simulink model "PTC_MBDS_ScrollCenteredNoWrap_Sample"  (R2013a)
settings: Solver=VariableStepDiscrete  StartTime=0.0  StopTime=100  RelTol=1e-3
undefined symbols (not defined in the file): sigbuilder_block
libraries: simulink_extras x1, PTC_MBDS_LIB x1
Description:
  | MBDS example or test model
settings Model: Creator=uid60719  LastModifiedBy=sundeep.tuteja
settings DataIOCC: LimitDataPoints=off  SignalLoggingSaveFormat=ModelDataLogs  SaveOutput=off  SignalLogging=off  SaveTime=off
settings OptimizationCC: ExpressionDepthLimit=2147483647  InitFltsAndDblsToZero=on
settings DebuggingCC: SaveWithParameterizedLinksMsg=none  SignalResolutionControl=TryResolveAllWithWarning  SolverPrmCheckMsg=none  InheritedTsInSrcMsg=none  DiscreteInheritContinuousMsg=none  MultiTaskDSMMsg=warning  MultiTaskCondExecSysMsg=none  FcnCallInpInsideContextMsg=UseLocalSettings  StrictBusMsg=Warning
settings RTWCC: IncludeERTFirstTime=on
settings GRTTargetCC: TargetFcnLib=ansi_tfl_tmw.mat  CombineOutputUpdateFcns=off  GRTInterface=on

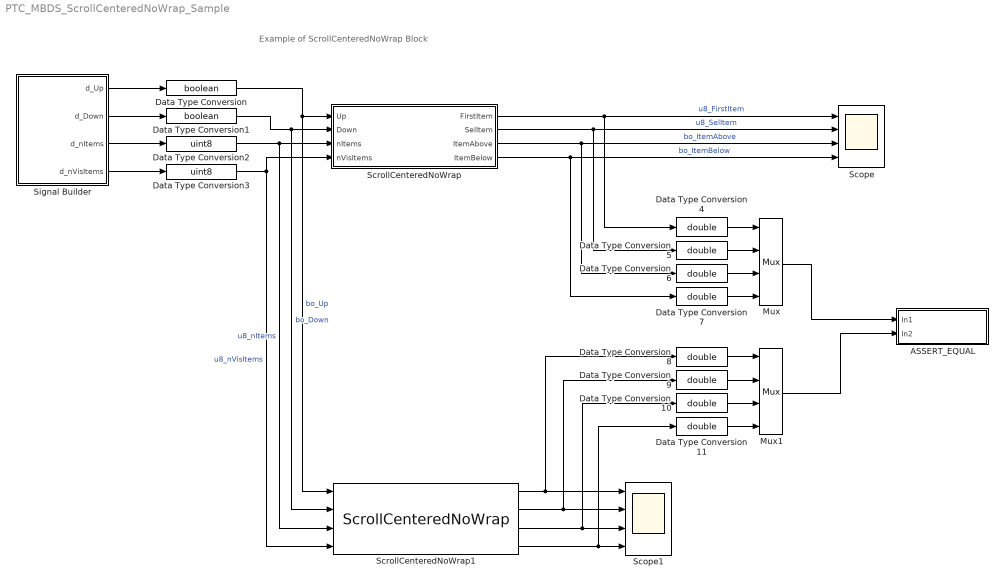
== system PTC_MBDS_ScrollCenteredNoWrap_Sample ==
  note: Example of ScrollCenteredNoWrap Block
  ASSERT_EQUAL : Subsystem
  Data Type Conversion : DataTypeConversion  OutDataTypeStr=boolean
      settings: MoveFcn=UpdateBlockSize(gcb);
  Data Type Conversion1 : DataTypeConversion  OutDataTypeStr=boolean
      settings: MoveFcn=UpdateBlockSize(gcb);
  Data Type Conversion2 : DataTypeConversion  OutDataTypeStr=uint8
      settings: MoveFcn=UpdateBlockSize(gcb);
  Data Type Conversion3 : DataTypeConversion  OutDataTypeStr=uint8
      settings: MoveFcn=UpdateBlockSize(gcb);
  Data Type Conversion{4..11} (8 alike) : DataTypeConversion  OutDataTypeStr=double
  Mux : Mux
  Mux1 : Mux
  Scope : Scope  NumInputPorts=4
      settings: YMin=-5~-5~-5~-5  YMax=5~5~5~5
  Scope1 : Scope  NumInputPorts=4
      settings: YMin=-5~-5~-5~-5  YMax=5~5~5~5
  ScrollCenteredNoWrap : Subsystem  InitFcn=|  mask(ScrollCenteredNoWrap){MBDS_LibraryBlock=on, MBDS_BlockVersion=05.40}
      | if(exist('MBDS_BlockCallback', 'file'))
      |    MBDS_BlockCallback('Update', gcb);
      | end
      mask prompts: MBDS_LibraryBlock "MBDS Library Block"; MBDS_BlockVersion "Block version:"
      mask help: Scroll within a list box and provide a centered selected/highlighted item. There is no roundtrip or wrap around at the beginning or end of the list.
      mask init:
      | if(exist('MBDS_BlockCallback', 'file'))
      |    MBDS_BlockCallback('Copy', gcb);
      | end
      mask Help: eval(['open([workdir(''Library_Dir:''),''\Blockset\Help\'',get_param(gcb,''MaskType''),''.html''])'])
      mask Display: disp(sprintf('Scroll\nCentered\nNo Wrap'))
  ScrollCenteredNoWrap1 : PTC_MBDS_LIB/MBDS Standard Library/Extended Operations/HMI/ScrollCenteredNoWrap  PTC_MBDS_BlockVersion=5.32  PTC_BlockType=PTC_MBDS_ScrollCenteredNoWrap
  Signal Builder : Subsystem  Tag=STV Subsys  LoadFcn=sigbuilder_block('load');  StartFcn=sigbuilder_block('start');  StopFcn=sigbuilder_block('stop');  ClipboardFcn=sigbuilder_block('clipboard');  mask(Sigbuilder block){}
      mask help: Create and generate interchangeable groups of signals whose waveforms are piecewise linear.
      mask init:
      | if ~strcmp(get_param(bdroot(gcbh),'SimulationStatus'),'stopped') tuvar = sigbuilder_block('maskInit'); end
      settings: CopyFcn=sigbuilder_block('copy');  DeleteFcn=sigbuilder_block('delete');  ModelCloseFcn=sigbuilder_block('modelClose');  PreSaveFcn=sigbuilder_block('preSave');  PauseFcn=sigbuilder_block('pause')  ContinueFcn=sigbuilder_block('continue')  NameChangeFcn=sigbuilder_block('namechange');  OpenFcn=sigbuilder_block('open',[78.75 74.25 550.5 399.75 ]);  CloseFcn=sigbuilder_block('close');
      mask Display: plot(0,0,100,100,[10,10,40,40,10],[80,20,20,80,80],[40,10],[50,50], [40,27,10],[65,72,56],[40,25,25,10],[28,28,43,43]);
  wires:
  Signal Builder/1(d_Up) -> Data Type Conversion/1
  Signal Builder/2(d_Down) -> Data Type Conversion1/1
  Signal Builder/3(d_nItems) -> Data Type Conversion2/1
  Signal Builder/4(d_nVisItems) -> Data Type Conversion3/1
  Data Type Conversion/1 -> ScrollCenteredNoWrap/1(Up), ScrollCenteredNoWrap1/1  "bo_Up"
  Data Type Conversion1/1 -> ScrollCenteredNoWrap/2(Down), ScrollCenteredNoWrap1/2  "bo_Down"
  Data Type Conversion2/1 -> ScrollCenteredNoWrap/3(nItems), ScrollCenteredNoWrap1/3  "u8_nItems"
  Data Type Conversion3/1 -> ScrollCenteredNoWrap/4(nVisItems), ScrollCenteredNoWrap1/4  "u8_nVisItems"
  ScrollCenteredNoWrap/1(FirstItem) -> Data Type Conversion4/1, Scope/1  "u8_FirstItem"
  ScrollCenteredNoWrap/2(SelItem) -> Data Type Conversion5/1, Scope/2  "u8_SelItem"
  ScrollCenteredNoWrap/3(ItemAbove) -> Data Type Conversion6/1, Scope/3  "bo_ItemAbove"
  ScrollCenteredNoWrap/4(ItemBelow) -> Data Type Conversion7/1, Scope/4  "bo_ItemBelow"
  ScrollCenteredNoWrap1/2 -> Scope1/2, Data Type Conversion9/1
  ScrollCenteredNoWrap1/1 -> Scope1/1, Data Type Conversion8/1
  ScrollCenteredNoWrap1/3 -> Data Type Conversion10/1, Scope1/3
  ScrollCenteredNoWrap1/4 -> Scope1/4, Data Type Conversion11/1
  Data Type Conversion4/1 -> Mux/1
  Data Type Conversion5/1 -> Mux/2
  Data Type Conversion6/1 -> Mux/3
  Data Type Conversion7/1 -> Mux/4
  Data Type Conversion8/1 -> Mux1/1
  Data Type Conversion9/1 -> Mux1/2
  Data Type Conversion10/1 -> Mux1/3
  Data Type Conversion11/1 -> Mux1/4
  Mux/1 -> ASSERT_EQUAL/1(In1)
  Mux1/1 -> ASSERT_EQUAL/2(In2)

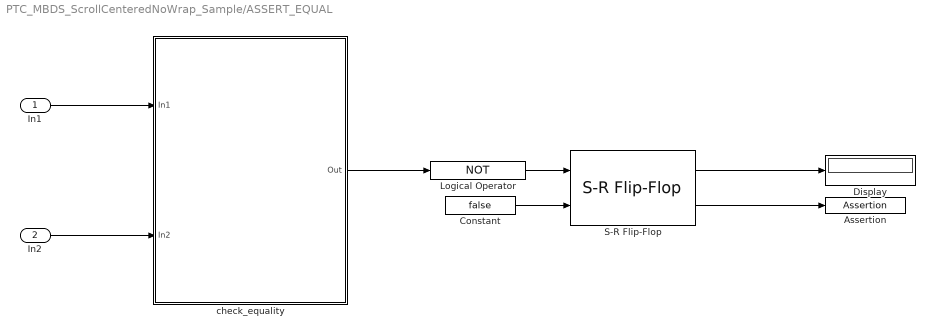
== system PTC_MBDS_ScrollCenteredNoWrap_Sample/ASSERT_EQUAL ==
  In1 : Inport
  In2 : Inport  Port=2
  Assertion : Assertion
  Constant : Constant  Value=false
  Display : Display
  Logical Operator : Logic  Operator=NOT  AllPortsSameDT=off  OutDataTypeStr=boolean
  S-R Flip-Flop : simulink_extras/Flip Flops/S-R Flip-Flop  initial_condition=0
  check_equality : MATLAB Function  TreatAsAtomicUnit=on
  wires:
  S-R Flip-Flop/1 -> Display/1
  check_equality/1(Out) -> Logical Operator/1
  Constant/1 -> S-R Flip-Flop/2
  S-R Flip-Flop/2 -> Assertion/1
  In2/1 -> check_equality/2(In2)
  In1/1 -> check_equality/1(In1)
  Logical Operator/1 -> S-R Flip-Flop/1

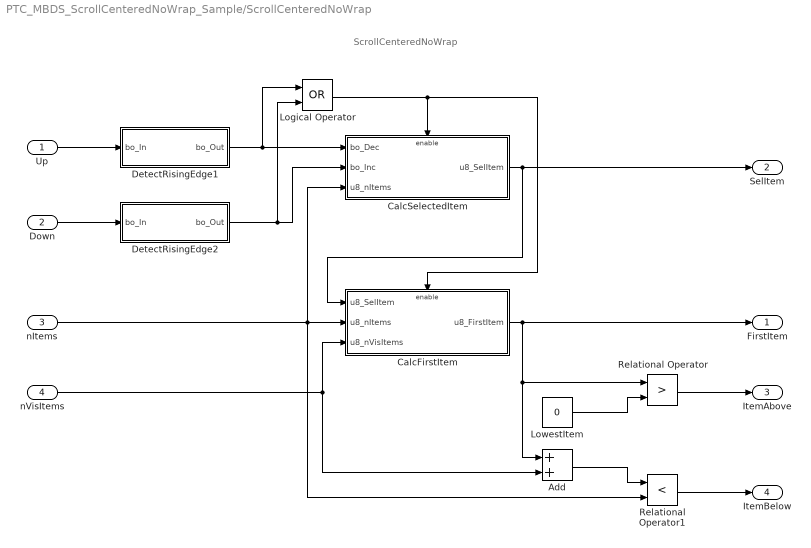
== system PTC_MBDS_ScrollCenteredNoWrap_Sample/ScrollCenteredNoWrap ==
  note: ScrollCenteredNoWrap
  Up : Inport  OutDataTypeStr=boolean  PortDimensions=1
  Down : Inport  Port=2  OutDataTypeStr=boolean  PortDimensions=1
  nItems : Inport  Port=3  OutDataTypeStr=uint8  PortDimensions=1
  nVisItems : Inport  Port=4  OutDataTypeStr=uint8  PortDimensions=1
  Add : Sum
  CalcFirstItem : Subsystem  TreatAsAtomicUnit=on
  CalcSelectedItem : Subsystem  TreatAsAtomicUnit=on
  DetectRisingEdge1 : Subsystem
  DetectRisingEdge2 : Subsystem
  Logical Operator : Logic  Operator=OR  AllPortsSameDT=off  OutDataTypeStr=boolean
  LowestItem : Constant  Value=0  OutDataTypeStr=uint8
  Relational Operator : RelationalOperator  Operator=>  OutDataTypeStr=boolean
  Relational Operator1 : RelationalOperator  Operator=<  OutDataTypeStr=boolean
  FirstItem : Outport  OutDataTypeStr=uint8  PortDimensions=1
  SelItem : Outport  Port=2  OutDataTypeStr=uint8  PortDimensions=1
  ItemAbove : Outport  Port=3  OutDataTypeStr=boolean  PortDimensions=1
  ItemBelow : Outport  Port=4  OutDataTypeStr=boolean  PortDimensions=1
  wires:
  Up/1 -> DetectRisingEdge1/1(bo_In)
  Down/1 -> DetectRisingEdge2/1(bo_In)
  CalcFirstItem/1(u8_FirstItem) -> Add/1, Relational Operator/1, FirstItem/1
  Relational Operator/1 -> ItemAbove/1
  Relational Operator1/1 -> ItemBelow/1
  CalcSelectedItem/1(u8_SelItem) -> SelItem/1, CalcFirstItem/1(u8_SelItem)
  Logical Operator/1 -> CalcSelectedItem/Enable, CalcFirstItem/Enable
  Add/1 -> Relational Operator1/1
  nItems/1 -> Relational Operator1/2, CalcFirstItem/2(u8_nItems), CalcSelectedItem/3(u8_nItems)
  DetectRisingEdge2/1(bo_Out) -> CalcSelectedItem/2(bo_Inc), Logical Operator/2
  DetectRisingEdge1/1(bo_Out) -> CalcSelectedItem/1(bo_Dec), Logical Operator/1
  nVisItems/1 -> CalcFirstItem/3(u8_nVisItems), Add/2
  LowestItem/1 -> Relational Operator/2

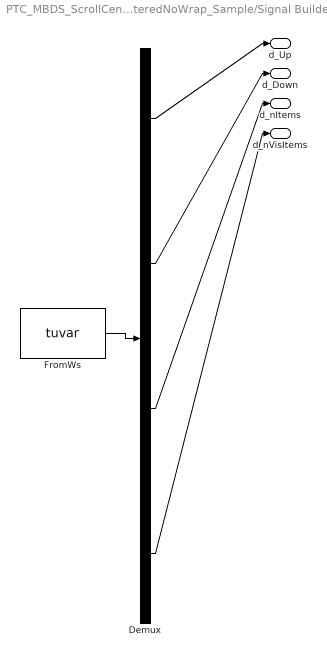
== system PTC_MBDS_ScrollCenteredNoWrap_Sample/Signal Builder ==
  Demux : Demux  Tag=STV Demux
  FromWs : FromWorkspace  Tag=STV FromWs  VariableName=tuvar  SampleTime=0
      SigBuilderData=|
      | common.afterFinalStr = 'Extrapolate'
      | common.sampleTime = 0
      | dataSet(1).timeRange = [0 10]
      | dataSet(1).name = 'TC1'
      | dataSet(2).timeRange = [0 10]
      | dataSet(2).name = 'TC2'
      | dataSet(3).timeRange = [0 10]
      | dataSet(3).name = 'TC3'
      | sbobj.Groups(1).Name = 'TC1'
      | sbobj.Groups(1).Signals(1).Name = 'd_Up'
      | sbobj.Groups(1).Signals(1).XData = [0 5.4 5.4 5.8 5.8 6 6 6.4 6.4 6.6 6.6 7 7 7.2 7.2 7.6 7.6 7.8 7.8 8.2 8.2 8.4 8.4 8.8 8.8 9 9 9.4 9.4 9.6 9.6 10]
      | sbobj.Groups(1).Signals(1).YData = [0 0 1 1 0 0 1 1 0 0 1 1 0 0 1 1 0 0 1 1 0 0 1 1 0 0 1 1 0 0 1 1]
      | sbobj.Groups(1).Signals(2).Name = 'd_Down'
      | sbobj.Groups(1).Signals(2).XData = [0 0.6 0.6 1 1 1.2 1.2 1.6 1.6 1.8 1.8 2.2 2.2 2.4 2.4 2.8 2.8 3 3 3.4 3.4 3.6 3.6 4 4 4.2 4.2 4.6 4.6 4.8 4.8 5.2 5.2 10]
      | sbobj.Groups(1).Signals(2).YData = [0 0 1 1 0 0 1 1 0 0 1 1 0 0 1 1 0 0 1 1 0 0 1 1 0 0 1 1 0 0 1 1 0 0]
      | sbobj.Groups(1).Signals(3).Name = 'd_nItems'
      | sbobj.Groups(1).Signals(3).XData = [0 10]
      | sbobj.Groups(1).Signals(3).YData = [6 6]
      | sbobj.Groups(1).Signals(4).Name = 'd_nVisItems'
      | sbobj.Groups(1).Signals(4).XData = [0 10]
      | sbobj.Groups(1).Signals(4).YData = [3 3]
      | sbobj.Groups(2).Name = 'TC2'
      | sbobj.Groups(2).Signals(1).Name = 'd_Up'
      | sbobj.Groups(2).Signals(1).XData = [0 5.4 5.4 5.8 5.8 6 6 6.4 6.4 6.6 6.6 7 7 7.2 7.2 7.6 7.6 7.8 7.8 8.2 8.2 8.4 8.4 8.8 8.8 9 9 9.4 9.4 9.6 9.6 10]
      | sbobj.Groups(2).Signals(1).YData = [0 0 1 1 0 0 1 1 0 0 1 1 0 0 1 1 0 0 1 1 0 0 1 1 0 0 1 1 0 0 1 1]
      | sbobj.Groups(2).Signals(2).Name = 'd_Down'
      | sbobj.Groups(2).Signals(2).XData = [0 0.6 0.6 1 1 1.2 1.2 1.6 1.6 1.8 1.8 2.2 2.2 2.4 2.4 2.8 2.8 3 3 3.4 3.4 3.6 3.6 4 4 4.2 4.2 4.6 4.6 4.8 4.8 5.2 5.2 10]
      | sbobj.Groups(2).Signals(2).YData = [0 0 1 1 0 0 1 1 0 0 1 1 0 0 1 1 0 0 1 1 0 0 1 1 0 0 1 1 0 0 1 1 0 0]
      | sbobj.Groups(2).Signals(3).Name = 'd_nItems'
      | sbobj.Groups(2).Signals(3).XData = [0 10]
      | sbobj.Groups(2).Signals(3).YData = [6 6]
      | sbobj.Groups(2).Signals(4).Name = 'd_nVisItems'
      | sbobj.Groups(2).Signals(4).XData = [0 10]
      | sbobj.Groups(2).Signals(4).YData = [4 4]
      | sbobj.Groups(3).Name = 'TC3'
      | sbobj.Groups(3).Signals(1).Name = 'd_Up'
      | sbobj.Groups(3).Signals(1).XData = [0 5.4 5.4 5.8 5.8 6 6 6.4 6.4 6.6 6.6 7 7 7.2 7.2 7.6 7.6 7.8 7.8 8.2 8.2 8.4 8.4 8.8 8.8 9 9 9.4 9.4 9.6 9.6 10]
      | sbobj.Groups(3).Signals(1).YData = [0 0 1 1 0 0 1 1 0 0 1 1 0 0 1 1 0 0 1 1 0 0 1 1 0 0 1 1 0 0 1 1]
      | sbobj.Groups(3).Signals(2).Name = 'd_Down'
      | sbobj.Groups(3).Signals(2).XData = [0 0.6 0.6 1 1 1.2 1.2 1.6 1.6 1.8 1.8 2.2 2.2 2.4 2.4 2.8 2.8 3 3 3.4 3.4 3.6 3.6 4 4 4.2 4.2 4.6 4.6 4.8 4.8 5.2 5.2 10]
      | sbobj.Groups(3).Signals(2).YData = [0 0 1 1 0 0 1 1 0 0 1 1 0 0 1 1 0 0 1 1 0 0 1 1 0 0 1 1 0 0 1 1 0 0]
      | sbobj.Groups(3).Signals(3).Name = 'd_nItems'
      | sbobj.Groups(3).Signals(3).XData = [0 10]
      | sbobj.Groups(3).Signals(3).YData = [6 6]
      | sbobj.Groups(3).Signals(4).Name = 'd_nVisItems'
      | sbobj.Groups(3).Signals(4).XData = [0 10]
      | sbobj.Groups(3).Signals(4).YData = [0 0]
  d_Up : Outport  Tag=STV Outport
  d_Down : Outport  Tag=STV Outport  Port=2
  d_nItems : Outport  Tag=STV Outport  Port=3
  d_nVisItems : Outport  Tag=STV Outport  Port=4
  wires:
  Demux/4 -> d_nVisItems/1
  Demux/3 -> d_nItems/1
  Demux/2 -> d_Down/1
  Demux/1 -> d_Up/1
  FromWs/1 -> Demux/1

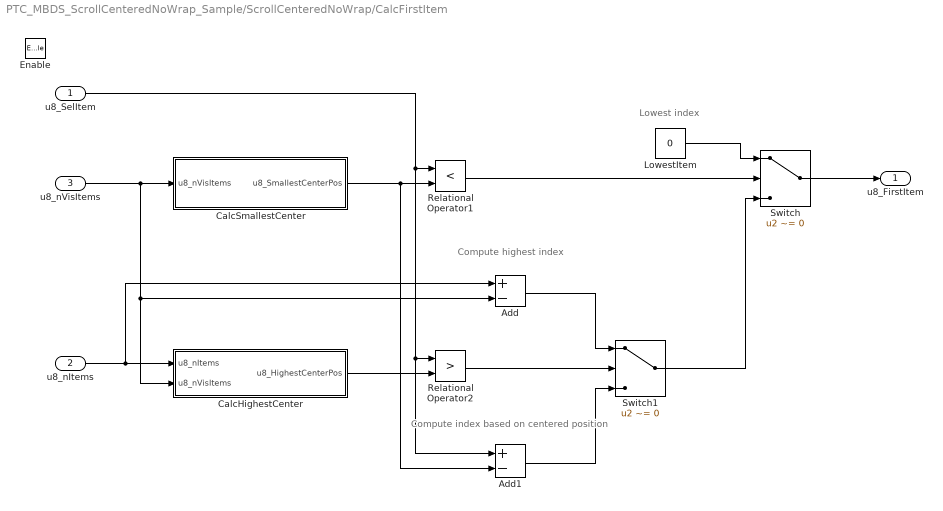
== system PTC_MBDS_ScrollCenteredNoWrap_Sample/ScrollCenteredNoWrap/CalcFirstItem ==
  note: Compute index based
      | on centered position
  note: Compute
      | highest index
  note: Lowest index
  u8_SelItem : Inport  OutDataTypeStr=uint8
  u8_nItems : Inport  Port=2  OutDataTypeStr=uint8
  u8_nVisItems : Inport  Port=3  OutDataTypeStr=uint8
  Enable : EnablePort
  Add : Sum  Inputs=+-
  Add1 : Sum  Inputs=+-
  CalcHighestCenter : Subsystem
  CalcSmallestCenter : Subsystem
  LowestItem : Constant  Value=0  OutDataTypeStr=uint8
  Relational Operator1 : RelationalOperator  Operator=<  OutDataTypeStr=boolean  InputSameDT=on
  Relational Operator2 : RelationalOperator  Operator=>  OutDataTypeStr=boolean  InputSameDT=on
  Switch : Switch  Criteria=u2 ~= 0  Threshold=0.5  OutDataTypeStr=Inherit: Inherit via back propagation  SaturateOnIntegerOverflow=on  InputSameDT=on
  Switch1 : Switch  Criteria=u2 ~= 0  Threshold=0.5  OutDataTypeStr=Inherit: Inherit via back propagation  SaturateOnIntegerOverflow=on  InputSameDT=on
  u8_FirstItem : Outport
  wires:
  u8_nVisItems/1 -> CalcSmallestCenter/1(u8_nVisItems), CalcHighestCenter/2(u8_nVisItems), Add/2
  u8_nItems/1 -> CalcHighestCenter/1(u8_nItems), Add/1
  CalcSmallestCenter/1(u8_SmallestCenterPos) -> Relational Operator1/2, Add1/2
  u8_SelItem/1 -> Relational Operator1/1, Relational Operator2/1, Add1/1
  CalcHighestCenter/1(u8_HighestCenterPos) -> Relational Operator2/2
  Switch/1 -> u8_FirstItem/1
  Relational Operator1/1 -> Switch/2
  Relational Operator2/1 -> Switch1/2
  Switch1/1 -> Switch/3
  Add/1 -> Switch1/1
  Add1/1 -> Switch1/3
  LowestItem/1 -> Switch/1

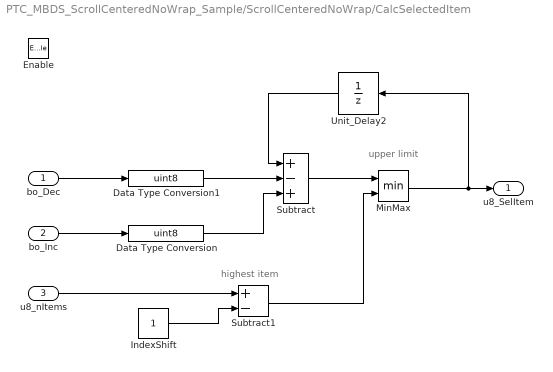
== system PTC_MBDS_ScrollCenteredNoWrap_Sample/ScrollCenteredNoWrap/CalcSelectedItem ==
  note: highest item
  note: upper limit
  bo_Dec : Inport  OutDataTypeStr=boolean
  bo_Inc : Inport  Port=2  OutDataTypeStr=boolean
  u8_nItems : Inport  Port=3  OutDataTypeStr=uint8
  Enable : EnablePort
  Data Type Conversion : DataTypeConversion  OutDataTypeStr=uint8
  Data Type Conversion1 : DataTypeConversion  OutDataTypeStr=uint8
  IndexShift : Constant  OutDataTypeStr=uint8
  MinMax : MinMax  Inputs=2  SaturateOnIntegerOverflow=on  InputSameDT=on
  Subtract : Sum  Inputs=+-+  AccumDataTypeStr=uint8  OutDataTypeStr=uint8  SaturateOnIntegerOverflow=on  InputSameDT=on
  Subtract1 : Sum  Inputs=+-  AccumDataTypeStr=uint8  OutDataTypeStr=Inherit: Inherit via back propagation
  Unit_Delay2 : UnitDelay  SampleTime=-1
      settings: AttributesFormatString=Init = %<X0>
  u8_SelItem : Outport
  wires:
  Subtract1/1 -> MinMax/2
  u8_nItems/1 -> Subtract1/1
  IndexShift/1 -> Subtract1/2
  bo_Inc/1 -> Data Type Conversion/1
  bo_Dec/1 -> Data Type Conversion1/1
  Data Type Conversion/1 -> Subtract/3
  Data Type Conversion1/1 -> Subtract/2
  Unit_Delay2/1 -> Subtract/1
  Subtract/1 -> MinMax/1
  MinMax/1 -> u8_SelItem/1, Unit_Delay2/1

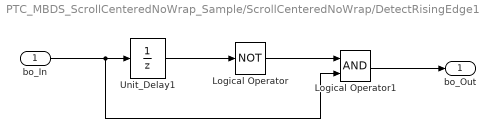
== system PTC_MBDS_ScrollCenteredNoWrap_Sample/ScrollCenteredNoWrap/DetectRisingEdge1 ==
  bo_In : Inport
  Logical Operator : Logic  Operator=NOT  OutDataTypeStr=boolean
  Logical Operator1 : Logic  OutDataTypeStr=boolean
  Unit_Delay1 : UnitDelay  SampleTime=-1
      settings: AttributesFormatString=Init = %<X0>
  bo_Out : Outport  PortDimensions=1
  wires:
  Logical Operator/1 -> Logical Operator1/1
  Unit_Delay1/1 -> Logical Operator/1
  Logical Operator1/1 -> bo_Out/1
  bo_In/1 -> Unit_Delay1/1, Logical Operator1/2

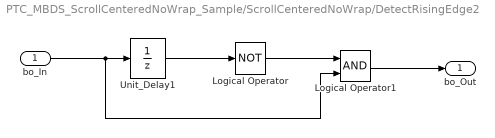
== system PTC_MBDS_ScrollCenteredNoWrap_Sample/ScrollCenteredNoWrap/DetectRisingEdge2 ==
  bo_In : Inport
  Logical Operator : Logic  Operator=NOT  OutDataTypeStr=boolean
  Logical Operator1 : Logic  OutDataTypeStr=boolean
  Unit_Delay1 : UnitDelay  SampleTime=-1
      settings: AttributesFormatString=Init = %<X0>
  bo_Out : Outport  PortDimensions=1
  wires:
  Logical Operator/1 -> Logical Operator1/1
  Unit_Delay1/1 -> Logical Operator/1
  Logical Operator1/1 -> bo_Out/1
  bo_In/1 -> Unit_Delay1/1, Logical Operator1/2

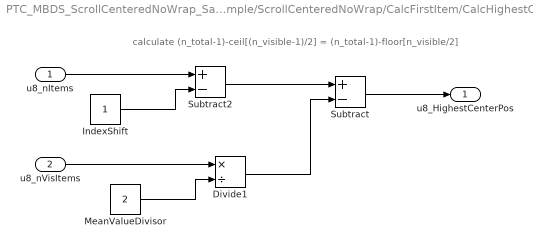
== system PTC_MBDS_ScrollCenteredNoWrap_Sample/ScrollCenteredNoWrap/CalcFirstItem/CalcHighestCenter ==
  note: calculate (n_total-1)-ceil[(n_visible-1)/2] = (n_total-1)-floor[n_visible/2]
  u8_nItems : Inport  OutDataTypeStr=uint8
  u8_nVisItems : Inport  Port=2  OutDataTypeStr=uint8
  Divide1 : Product  Inputs=*/  OutDataTypeStr=uint8
  IndexShift : Constant  OutDataTypeStr=uint8
  MeanValueDivisor : Constant  Value=2  OutDataTypeStr=uint8
  Subtract : Sum  Inputs=+-  OutDataTypeStr=uint8  InputSameDT=on
  Subtract2 : Sum  Inputs=+-  OutDataTypeStr=uint8  InputSameDT=on
  u8_HighestCenterPos : Outport
  wires:
  u8_nVisItems/1 -> Divide1/1
  Divide1/1 -> Subtract/2
  Subtract/1 -> u8_HighestCenterPos/1
  u8_nItems/1 -> Subtract2/1
  Subtract2/1 -> Subtract/1
  IndexShift/1 -> Subtract2/2
  MeanValueDivisor/1 -> Divide1/2

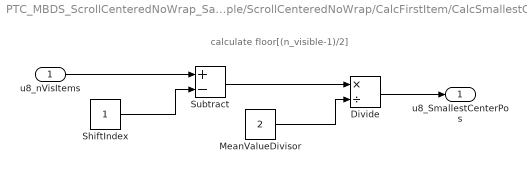
== system PTC_MBDS_ScrollCenteredNoWrap_Sample/ScrollCenteredNoWrap/CalcFirstItem/CalcSmallestCenter ==
  note: calculate floor[(n_visible-1)/2]
  u8_nVisItems : Inport  OutDataTypeStr=uint8
  Divide : Product  Inputs=*/  OutDataTypeStr=uint8
  MeanValueDivisor : Constant  Value=2  OutDataTypeStr=uint8
  ShiftIndex : Constant  OutDataTypeStr=uint8
  Subtract : Sum  Inputs=+-  OutDataTypeStr=uint8  InputSameDT=on
  u8_SmallestCenterPos : Outport
  wires:
  u8_nVisItems/1 -> Subtract/1
  Subtract/1 -> Divide/1
  Divide/1 -> u8_SmallestCenterPos/1
  ShiftIndex/1 -> Subtract/2
  MeanValueDivisor/1 -> Divide/2

== matlab function PTC_MBDS_ScrollCenteredNoWrap_Sample/ASSERT_EQUAL/check_equality ==
  data: In1 input; Out output; In2 input
function Out = check_equality(In1, In2)
%#codegen

Out = isequaln(In1, In2);

end
